simulink model "PENDULO_CARRO_NO_LINEAL"  (R2018a)
settings: Solver=ode4  StartTime=0.0  StopTime=100  FixedStep=0.0001  RelTol=1e-3
undefined symbols (not defined in the file or in its folder): P10, P2, P3, P4, P5, P7, P8, P9
libraries: dspinverses x1
settings Model: Creator=Omie-PC  LastModifiedBy=Benjamin Nicolas

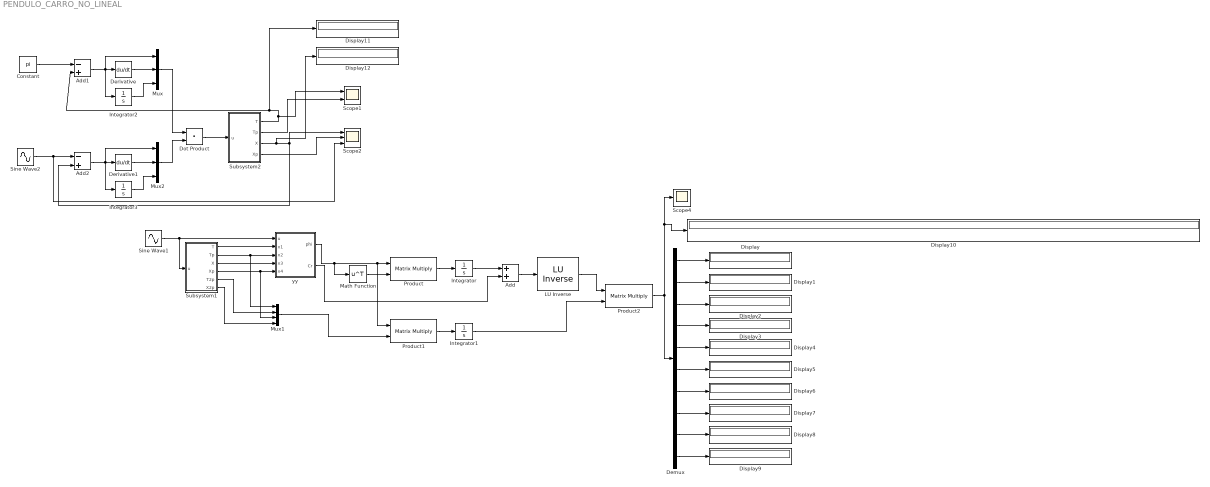
== system PENDULO_CARRO_NO_LINEAL ==
  " LU Inverse" : dspinverses/ LU Inverse
      settings: SourceProductName=DSP System Toolbox
  Add : Sum
  Add1 : Sum  Inputs=-+
  Add2 : Sum  Inputs=-+
  Constant : Constant  Value=pi
  Demux : Demux  Outputs=10
  Derivative : Derivative
  Derivative1 : Derivative
  Display{,1..12} (13 alike) : Display
  Dot Product : DotProduct  InputSameDT=on  OutDataTypeStr=Inherit: Inherit via internal rule
  Integrator{,1..3} (4 alike) : Integrator
  Math Function : Math  Operator=transpose  SaturateOnIntegerOverflow=on
  Mux : Mux  Inputs=3
  Mux1 : Mux
  Mux2 : Mux  Inputs=3
  Product : Product  Multiplication=Matrix(*)
  Product1 : Product  Multiplication=Matrix(*)
  Product2 : Product  Multiplication=Matrix(*)
  Scope1 : Scope  NumInputPorts=2
  Scope2 : Scope  NumInputPorts=3
  Scope4 : Scope
  Sine Wave1 : Sin  Frequency=6000  SampleTime=0
  Sine Wave2 : Sin  Frequency=10000  SampleTime=0
  Subsystem1 : Subsystem
  Subsystem2 : Subsystem
  yy : MATLAB Function  TreatAsAtomicUnit=on
  wires:
  yy/2(Cr) -> Add/2
  Demux/5 -> Display4/1
  Product/1 -> Integrator/1
  Demux/3 -> Display2/1
  Demux/1 -> Display/1
  Product1/1 -> Integrator1/1
  " LU Inverse"/1 -> Product2/1
  yy/1(phi) -> Product1/1, Product/1, Math Function/1
  Demux/2 -> Display1/1
  Product2/1 -> Display10/1, Scope4/1, Demux/1
  Integrator1/1 -> Product2/2
  Demux/4 -> Display3/1
  Mux1/1 -> Product1/2
  Add/1 -> " LU Inverse"/1
  Math Function/1 -> Product/2
  Integrator/1 -> Add/1
  Sine Wave1/1 -> Subsystem1/1(u), yy/1(u)
  Demux/10 -> Display9/1
  Demux/9 -> Display8/1
  Demux/8 -> Display7/1
  Demux/7 -> Display6/1
  Demux/6 -> Display5/1
  Subsystem1/1(T) -> yy/2(x1)
  Subsystem1/2(Tp) -> Mux1/1, yy/3(x2)
  Subsystem1/3(X) -> yy/4(x3)
  Subsystem1/4(Xp) -> Mux1/3, yy/5(x4)
  Subsystem1/5(T2p) -> Mux1/2
  Subsystem1/6(X2p) -> Mux1/4
  Subsystem2/1(T) -> Display11/1, Add1/2, Scope1/1
  Subsystem2/2(Tp) -> Scope1/2
  Subsystem2/3(X) -> Display12/1, Scope2/1, Add2/2
  Subsystem2/4(Xp) -> Scope2/2
  Constant/1 -> Add1/1
  Add1/1 -> Mux/1, Integrator2/1, Derivative/1
  Derivative/1 -> Mux/2
  Integrator2/1 -> Mux/3
  Integrator3/1 -> Mux2/3
  Sine Wave2/1 -> Scope2/3, Add2/1
  Add2/1 -> Mux2/1, Integrator3/1, Derivative1/1
  Derivative1/1 -> Mux2/2
  Dot Product/1 -> Subsystem2/1(u)
  Mux2/1 -> Dot Product/2
  Mux/1 -> Dot Product/1

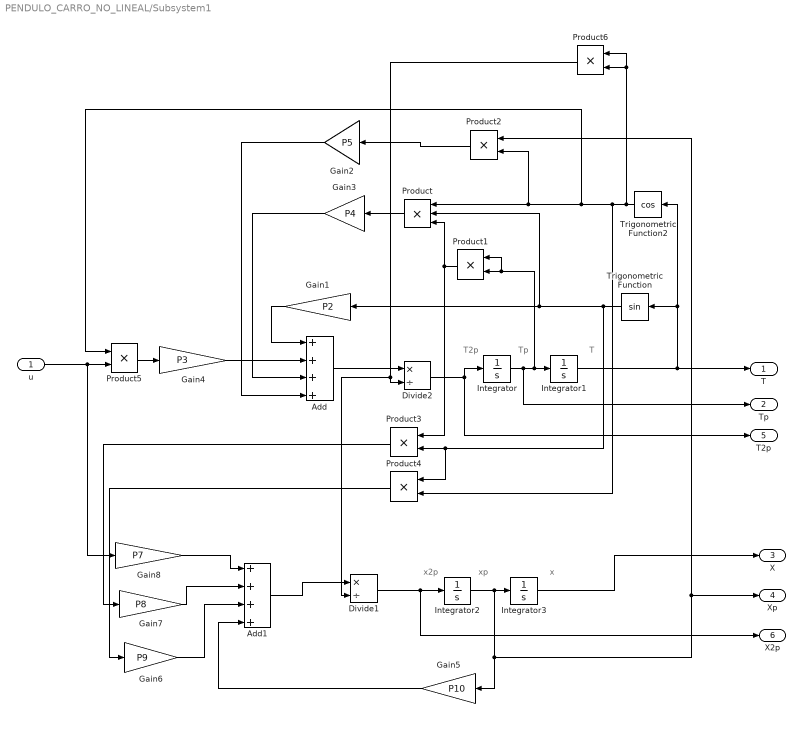
== system PENDULO_CARRO_NO_LINEAL/Subsystem1 ==
  note: x2p
  note: xp
  note: x
  note: T
  note: T2p
  note: Tp
  u : Inport
  Add : Sum  Inputs=++++
  Add1 : Sum  Inputs=++++
  Divide1 : Product  Inputs=*/
  Divide2 : Product  Inputs=*/
  Gain1 : Gain  Gain=P2
  Gain2 : Gain  Gain=P5
  Gain3 : Gain  Gain=P4
  Gain4 : Gain  Gain=P3
  Gain5 : Gain  Gain=P10
  Gain6 : Gain  Gain=P9
  Gain7 : Gain  Gain=P8
  Gain8 : Gain  Gain=P7
  Integrator : Integrator
  Integrator1 : Integrator  InitialCondition=pi
  Integrator2 : Integrator
  Integrator3 : Integrator
  Product : Product  Inputs=3
  Product{1..6} (6 alike) : Product
  Trigonometric Function : Trigonometry
  Trigonometric Function2 : Trigonometry  Operator=cos
  T : Outport
  Tp : Outport  Port=2
  X : Outport  Port=3
  Xp : Outport  Port=4
  T2p : Outport  Port=5
  X2p : Outport  Port=6
  wires:
  Integrator3/1 -> X/1
  Product/1 -> Gain3/1
  Gain5/1 -> Add1/4
  Gain3/1 -> Add/3
  Integrator2/1 -> Integrator3/1, Gain5/1, Product2/1, Xp/1
  Gain2/1 -> Add/4
  Product3/1 -> Gain7/1
  Gain7/1 -> Add1/2
  Gain8/1 -> Add1/1
  Gain6/1 -> Add1/3
  Gain1/1 -> Add/1
  Product4/1 -> Gain6/1
  Product2/1 -> Gain2/1
  Integrator/1 -> Tp/1, Product1/2, Product1/1, Integrator1/1
  Product1/1 -> Product/3, Product3/1
  Gain4/1 -> Add/2
  Trigonometric Function/1 -> Product/2, Gain1/1, Product3/2, Product4/1
  Integrator1/1 -> Trigonometric Function/1, Trigonometric Function2/1, T/1
  Product5/1 -> Gain4/1
  u/1 -> Gain8/1, Product5/2
  Trigonometric Function2/1 -> Product6/1, Product6/2, Product5/1, Product/1, Product2/2, Product4/2
  Add1/1 -> Divide1/1
  Divide1/1 -> X2p/1, Integrator2/1
  Add/1 -> Divide2/1
  Divide2/1 -> T2p/1, Integrator/1
  Product6/1 -> Divide1/2, Divide2/2

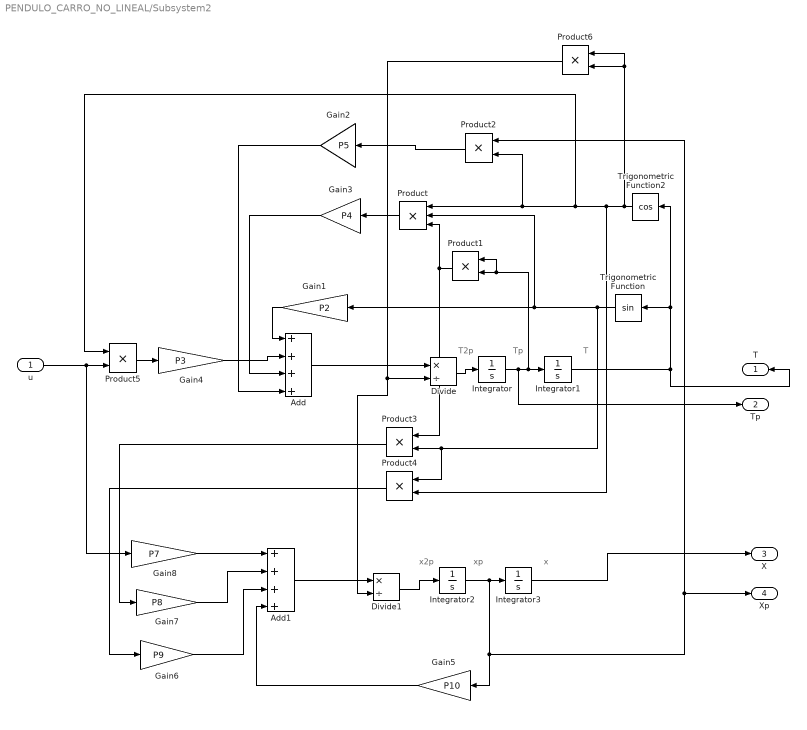
== system PENDULO_CARRO_NO_LINEAL/Subsystem2 ==
  note: Tp
  note: T2p
  note: T
  note: x
  note: xp
  note: x2p
  u : Inport
  Add : Sum  Inputs=++++
  Add1 : Sum  Inputs=++++
  Divide : Product  Inputs=*/
  Divide1 : Product  Inputs=*/
  Gain1 : Gain  Gain=P2
  Gain2 : Gain  Gain=P5
  Gain3 : Gain  Gain=P4
  Gain4 : Gain  Gain=P3
  Gain5 : Gain  Gain=P10
  Gain6 : Gain  Gain=P9
  Gain7 : Gain  Gain=P8
  Gain8 : Gain  Gain=P7
  Integrator : Integrator
  Integrator1 : Integrator  InitialCondition=pi
  Integrator2 : Integrator  InitialCondition=0.1
  Integrator3 : Integrator
  Product : Product  Inputs=3
  Product{1..6} (6 alike) : Product
  Trigonometric Function : Trigonometry
  Trigonometric Function2 : Trigonometry  Operator=cos
  T : Outport
  Tp : Outport  Port=2
  X : Outport  Port=3
  Xp : Outport  Port=4
  wires:
  u/1 -> Product5/2, Gain8/1
  Product5/1 -> Gain4/1
  Integrator1/1 -> T/1, Trigonometric Function2/1, Trigonometric Function/1
  Trigonometric Function/1 -> Product4/1, Product3/2, Gain1/1, Product/2
  Gain4/1 -> Add/2
  Product1/1 -> Product3/1, Product/3
  Integrator/1 -> Integrator1/1, Product1/1, Product1/2, Tp/1
  Product2/1 -> Gain2/1
  Product4/1 -> Gain6/1
  Gain1/1 -> Add/1
  Gain6/1 -> Add1/3
  Gain8/1 -> Add1/1
  Gain7/1 -> Add1/2
  Product3/1 -> Gain7/1
  Gain2/1 -> Add/4
  Integrator2/1 -> Xp/1, Product2/1, Gain5/1, Integrator3/1
  Gain3/1 -> Add/3
  Gain5/1 -> Add1/4
  Product/1 -> Gain3/1
  Integrator3/1 -> X/1
  Divide/1 -> Integrator/1
  Trigonometric Function2/1 -> Product6/1, Product6/2, Product4/2, Product2/2, Product/1, Product5/1
  Add/1 -> Divide/1
  Product6/1 -> Divide1/2, Divide/2
  Divide1/1 -> Integrator2/1
  Add1/1 -> Divide1/1

== matlab function PENDULO_CARRO_NO_LINEAL/yy ==
  data: u input; x1 input; phi output; x2 input; x3 input; Cr output; x4 input
function [phi,Cr]  = fcn(u,x1,x2,x3,x4)
k=0.1;
Cr=k*eye(10);
phi = [x2,0,0,0;0,sin(x1)/cos(x1)^2,0,0;0,u/cos(x1),0,0;0,x2^2*sin(x1)/cos(x1),0,0;0,x4/cos(x1),0,0;0,0,1,0;0,0,0,u/cos(x1)^2;0,0,0,x2^2*sin(x1)/cos(x1)^2;0,0,0,sin(x1)/cos(x1);0,0,0,x4/cos(x1)^2];
